simulink model "Microgrid_transition_model_092021"  (R2020a)
settings: Solver=VariableStepAuto  StartTime=0.0  StopTime=10  MaxStep=1e-4  RelTol=1e-3
PreLoadFcn:
  | %run('FC_microgrid_param.m')
  | %load('bat_grid_init.m')
InitFcn:
  | %load myisoModel_init;
  | run('FC_microgrid_param.m')
  | tic
  | run('CARTinitFcn.m')
  | %caseNo = 2;
  | 
  | %if (caseNo == 1)
  | %set_param(['Isolated_grid_paper_model_022521/SignalGen'], 'ActiveScenario', 'PStep222kW');
  | %else
  | %set_param(['Isolated_grid_paper_model_022521/SignalGen'], 'ActiveScenario', 'QStep222kVAr');
  | 
  | %end;
StopFcn:
  | toc
undefined symbols (not defined in the file): breakpoints1, breakpoints2, cp_table_data, ctrl, D1, D11, Delta, DiscIntNeverNeededParam, DT, FC_BESS, find_system, gcbh, libFC_BESS, LowerLimit, magnitude, oversize, pq_ts, sps_rtmsupport, timer, ts, Ts, Ts_APC, Ts_Control, Ts_Power, UpperLimit
libraries: powerlib x128, powerlib_meascontrol x81, simulink x63, powerlib_extras x40, simulink_extras x12, sps_avr x7, pi_ctrl x4, SignalEditorBlockLib x2, libLgBattery x1, libFC_PV x1, eePowerMeasurement x1, spsDieselMotorModel x1
(part 7 of 10)

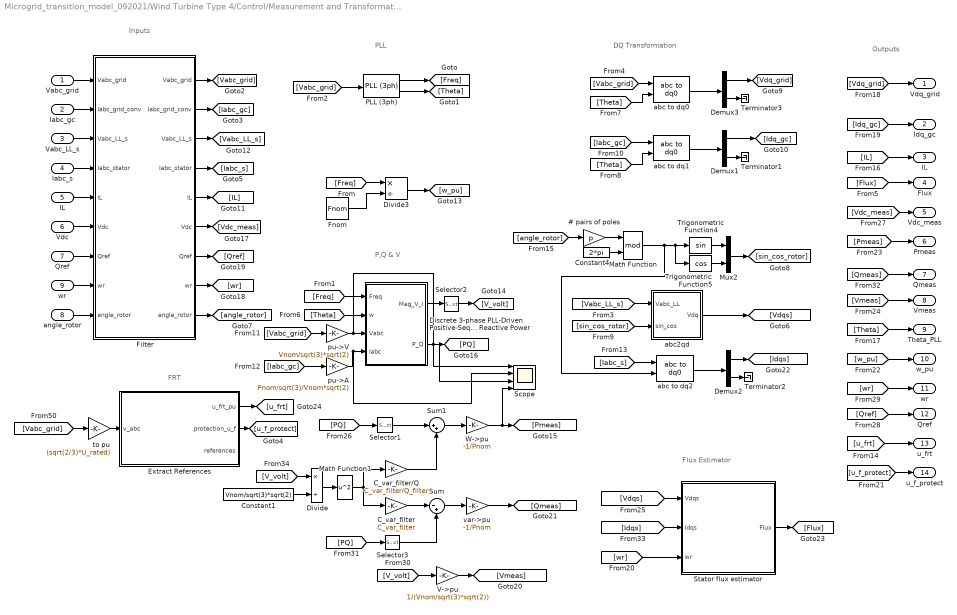
== system Microgrid_transition_model_092021/Wind Turbine Type 4/Control/Measurement and Transformation ==
  note: Flux Estimator
  note: Outputs
  note: PLL
  note: DQ Transformation
  note: P,Q & V
  note: Inputs
  note: FRT
  Vabc_grid : Inport
  Iabc_gc : Inport  Port=2
  Vabc_LL_s : Inport  Port=3
  Iabc_s : Inport  Port=4
  IL : Inport  Port=5
  Vdc : Inport  Port=6
  Qref : Inport  Port=7
  angle_rotor : Inport  Port=8
  wr : Inport  Port=9
  # pairs of poles : Gain  Gain=p  SaturateOnIntegerOverflow=on  OutDataTypeStr=Inherit: Same as input  ParamDataTypeStr=Inherit: Same as input
  C_var_filter : Gain  Gain=C_var_filter  SaturateOnIntegerOverflow=on  OutDataTypeStr=Inherit: Same as input  ParamDataTypeStr=Inherit: Same as input
  C_var_filter/Q : Gain  Gain=C_var_filter/Q_filter  SaturateOnIntegerOverflow=on  OutDataTypeStr=Inherit: Same as input  ParamDataTypeStr=Inherit: Same as input
  Constant1 : Constant  Value=Vnom/sqrt(3)*sqrt(2)
  Constant4 : Constant  Value=2*pi
  Demux1 : Demux  Outputs=[2 1]
      settings: DisplayOption=none
  Demux2 : Demux  Outputs=[2 1]
      settings: DisplayOption=none
  Demux3 : Demux  Outputs=[2 1]
      settings: DisplayOption=none
  Discrete 3-phase PLL-Driven Positive-Sequence Active & Reactive Power : Subsystem  mask(Discrete 3-phase PLL-Driven Positive-Sequence Active & Reactive Power){Finit=Fnom, Fmin=Fnom*45/60, Par_Vinit=[Vnom/sqrt(3)*sqrt(2) 30], Par_Iinit=[Pnom/sqrt(3)/Vnom*sqrt(2) -10], Ts=Ts}
      mask prompts: Finit "Initial frequency (Hz):"; Fmin "Minimum frequency (Hz):"; Par_Vinit "Voltage initial input: [ Mag  Phase(Degrees) ]"; Par_Iinit "Current initial input: [ Mag  Phase(Degrees) ]"; Ts "Sample time:"
      mask help:
      | This discrete block measures the 3-phase active power P and reactive power Q  associated with a periodic set of 3-phase voltages and currents which may contain harmonics. P and Q are calculated by evaluating the fundamental values (positive-sequence) of the input voltages and currents with a running window over one cycle of the specified frequency (port Freq).
      |  Input port "Sin_Cos" (a two-dimension signal) provides the reference frame required for the computation.
      |
      | input 1: must give the frequency of the fundamental (Hz)
      | Input 2: must contain a  [sin(wt)  cos(wt)] two dimension signal , where w is the rotation speed (rad/s) of the reference frame used for the computation..
      | input 3: Vectorized 3-phase  instantaneous voltage (Vabc)
      | input 4: Vectorized 3-phase instantaneous current (Iabc)
      |
      | Output 1: Vector [Mag_V Mag_I] of the fundamental values (Magnitude) of the voltage & current (peak values of the positive-sequence)
      | Output 2: 3-phase PQ measurement vector [P(W) Q (var)] evaluated at the specified frequency. Current flowing into an RL circuit will produce  positive active and reactive powers.
      |
      | For the first cycle of simulation, the outputs are held constant using the values specified by the parameters "Initial input".
      | he value of the parameter "Minimum frequency" is used to determine the buffer size of the "Variable Transport Delay" block found inside this subsystem.
      mask init:
      | power_initmask();
      settings: OpenFcn=power_openblockproxy();
  Divide : Product  Inputs=*/
  Divide3 : Product  Inputs=*/
  Extract References : Subsystem
  Filter : Subsystem  mask{Freq=Freq_filter, Zeta=Zeta_filter, Ts=Ts}
      mask prompts: Freq "Cut-off frequency (Hz):"; Zeta "Damping factor Zeta:"; Ts "Sample time"
  Fnom : Constant  Value=Fnom
  Math Function : Math  Operator=mod  SignedPower=on  SaturateOnIntegerOverflow=on
  Math Function1 : Math  Operator=square  SignedPower=on  SaturateOnIntegerOverflow=on
  Mux2 : Mux  Inputs=2
  PLL (3ph) : powerlib_meascontrol/PLL/PLL (3ph)  Fmin=0.75*Fnom  Par_Init=[-45 Fnom]  ParK=[60 1400 1]  TcD=1e-4  MaxRateChangeFreq=12  FilterCutOffFreq=25  Ts=Ts  AGC=on
      settings: SourceProductBaseCode=MT,PS
  Scope : Scope  NumInputPorts=4
  Selector1 : Selector  InputPortWidth=2  IndexOptions=Index vector (dialog)  Indices=1  OutputSizes=1
  Selector2 : Selector  InputPortWidth=2  IndexOptions=Index vector (dialog)  Indices=1  OutputSizes=1
  Selector3 : Selector  InputPortWidth=2  IndexOptions=Index vector (dialog)  Indices=2  OutputSizes=1
  Stator flux estimator : Subsystem
  Sum : Sum  Inputs=|-+
  Sum1 : Sum  Inputs=|++
  Terminator1 : Terminator
  Terminator2 : Terminator
  Terminator3 : Terminator
  Trigonometric Function4 : Trigonometry
  Trigonometric Function5 : Trigonometry  Operator=cos
  V->pu : Gain  Gain=1/(Vnom/sqrt(3)*sqrt(2))  SaturateOnIntegerOverflow=on  OutDataTypeStr=Inherit: Same as input  ParamDataTypeStr=Inherit: Same as input
  W->pu : Gain  Gain=-1/Pnom  SaturateOnIntegerOverflow=on  OutDataTypeStr=Inherit: Same as input  ParamDataTypeStr=Inherit: Same as input
  abc to dq0 : powerlib_meascontrol/Transformations/abc to dq0  Alignment=90 degrees behind phase A axis
      settings: SourceProductBaseCode=MT,PS
  abc to dq1 : powerlib_meascontrol/Transformations/abc to dq0  Alignment=90 degrees behind phase A axis
      settings: SourceProductBaseCode=MT,PS
  abc to dq2 : powerlib_meascontrol/Transformations/abc to dq0  Alignment=90 degrees behind phase A axis
      settings: SourceProductBaseCode=MT,PS
  abc2qd : Subsystem
  pu->A : Gain  Gain=Pnom/sqrt(3)/Vnom*sqrt(2)  SaturateOnIntegerOverflow=on  OutDataTypeStr=Inherit: Same as input  ParamDataTypeStr=Inherit: Same as input
  pu->V : Gain  Gain=Vnom/sqrt(3)*sqrt(2)  SaturateOnIntegerOverflow=on  OutDataTypeStr=Inherit: Same as input  ParamDataTypeStr=Inherit: Same as input
  to pu : Gain  Gain=(sqrt(2/3)*U_rated)
  "var->pu " : Gain  Gain=-1/Pnom  SaturateOnIntegerOverflow=on  OutDataTypeStr=Inherit: Same as input  ParamDataTypeStr=Inherit: Same as input
  Vdq_grid : Outport  VectorParamsAs1DForOutWhenUnconnected=off
  Idq_gc : Outport  Port=2  VectorParamsAs1DForOutWhenUnconnected=off
  "IL " : Outport  Port=3  VectorParamsAs1DForOutWhenUnconnected=off
  Flux : Outport  Port=4  VectorParamsAs1DForOutWhenUnconnected=off
  Vdc_meas : Outport  Port=5  VectorParamsAs1DForOutWhenUnconnected=off
  Pmeas : Outport  Port=6  VectorParamsAs1DForOutWhenUnconnected=off
  Qmeas : Outport  Port=7  VectorParamsAs1DForOutWhenUnconnected=off
  Vmeas : Outport  Port=8  VectorParamsAs1DForOutWhenUnconnected=off
  Theta_PLL : Outport  Port=9  VectorParamsAs1DForOutWhenUnconnected=off
  w_pu : Outport  Port=10  VectorParamsAs1DForOutWhenUnconnected=off
  "wr " : Outport  Port=11  VectorParamsAs1DForOutWhenUnconnected=off
  "Qref " : Outport  Port=12  VectorParamsAs1DForOutWhenUnconnected=off
  u_frt : Outport  Port=13
  u_f_protect : Outport  Port=14
  wires:
  Filter/9("angle_rotor ") -> [angle_rotor]
  angle_rotor/1 -> Filter/9(angle_rotor)
  Stator flux estimator/1(Flux) -> [Flux]
  # pairs of poles/1 -> Math Function/1
  Constant4/1 -> Math Function/2
  abc2qd/1(Vdq) -> [Vdqs]
  Trigonometric Function5/1 -> Mux2/2
  Trigonometric Function4/1 -> Mux2/1
  [angle_rotor] -> # pairs of poles/1
  [Vabc_LL_s] -> abc2qd/1(Vabc_LL)
  [sin_cos_rotor] -> abc2qd/2(sin_cos)
  Mux2/1 -> [sin_cos_rotor]
  Demux2/1 -> [Idqs]
  Demux2/2 -> Terminator2/1
  abc to dq2/1 -> Demux2/1
  [Iabc_s] -> abc to dq2/1
  [Vdqs] -> Stator flux estimator/1(Vdqs)
  [Idqs] -> Stator flux estimator/2(Idqs)
  [wr] -> Stator flux estimator/3(wr)
  [Qmeas] -> Qmeas/1
  "var->pu "/1 -> [Qmeas]
  [PQ] -> Selector3/1
  V->pu/1 -> [Vmeas]
  [V_volt] -> V->pu/1
  Selector2/1 -> [V_volt]
  Discrete 3-phase PLL-Driven Positive-Sequence Active & Reactive Power/1(Mag_V_I) -> Selector2/1
  Demux1/2 -> Terminator1/1
  Demux3/1 -> [Vdq_grid]
  Demux3/2 -> Terminator3/1
  abc to dq1/1 -> Demux1/1
  abc to dq0/1 -> Demux3/1
  PLL (3ph)/1 -> [Freq]
  Fnom/1 -> Divide3/2
  Divide3/1 -> [w_pu]
  pu->V/1 -> Scope/1, Discrete 3-phase PLL-Driven Positive-Sequence Active & Reactive Power/3(Vabc)
  W->pu/1 -> Scope/4, [Pmeas]
  [Freq] -> Divide3/1
  [Freq] -> Discrete 3-phase PLL-Driven Positive-Sequence Active & Reactive Power/1(Freq)
  PLL (3ph)/2 -> [Theta]
  [Vabc_grid] -> abc to dq0/1
  [Theta] -> Discrete 3-phase PLL-Driven Positive-Sequence Active & Reactive Power/2(w)
  [Theta] -> abc to dq0/2
  [Theta] -> abc to dq1/2
  [Vabc_grid] -> PLL (3ph)/1
  [Iabc_gc] -> abc to dq1/1
  [Theta] -> Theta_PLL/1
  Demux1/1 -> [Idq_gc]
  [Vdq_grid] -> Vdq_grid/1
  [Idq_gc] -> Idq_gc/1
  [w_pu] -> w_pu/1
  [Pmeas] -> Pmeas/1
  [Vmeas] -> Vmeas/1
  pu->A/1 -> Discrete 3-phase PLL-Driven Positive-Sequence Active & Reactive Power/4(Iabc), Scope/2
  [PQ] -> Selector1/1
  [Vdc_meas] -> Vdc_meas/1
  [Qref] -> "Qref "/1
  [wr] -> "wr "/1
  [Flux] -> Flux/1
  [Vabc_grid] -> pu->V/1
  [Iabc_gc] -> pu->A/1
  Discrete 3-phase PLL-Driven Positive-Sequence Active & Reactive Power/2(P_Q) -> Scope/3, [PQ]
  Vabc_grid/1 -> Filter/1(Vabc_grid)
  Vdc/1 -> Filter/6(Vdc)
  Qref/1 -> Filter/7(Qref)
  wr/1 -> Filter/8(wr)
  Filter/1("Vabc_grid ") -> [Vabc_grid]
  Filter/2("Iabc_grid_conv ") -> [Iabc_gc]
  Filter/4("Iabc_stator ") -> [Iabc_s]
  Filter/6("Vdc ") -> [Vdc_meas]
  Filter/8("wr ") -> [wr]
  Filter/7("Qref ") -> [Qref]
  Iabc_gc/1 -> Filter/2(Iabc_grid_conv)
  Iabc_s/1 -> Filter/4(Iabc_stator)
  Vabc_LL_s/1 -> Filter/3(Vabc_LL_s)
  Filter/3("Vabc_LL_s ") -> [Vabc_LL_s]
  [V_volt] -> Divide/1
  Constant1/1 -> Divide/2
  Divide/1 -> Math Function1/1
  Selector3/1 -> Sum/2
  C_var_filter/1 -> Sum/1
  Sum/1 -> "var->pu "/1
  Math Function1/1 -> C_var_filter/Q/1, C_var_filter/1
  Selector1/1 -> Sum1/1
  C_var_filter/Q/1 -> Sum1/2
  Sum1/1 -> W->pu/1
  IL/1 -> Filter/5(IL)
  Filter/5("IL ") -> [IL]
  [IL] -> "IL "/1
  Math Function/1 -> abc to dq2/2, Trigonometric Function5/1, Trigonometric Function4/1
  Extract References/1(u_frt_pu) -> [u_frt]
  Extract References/2(protection_u_f) -> [u_f_protect]
  [Vabc_grid] -> to pu/1
  [u_frt] -> u_frt/1
  [u_f_protect] -> u_f_protect/1
  to pu/1 -> Extract References/1(v_abc)

== system Microgrid_transition_model_092021/Wind Turbine Type 4/Control/Speed & Pitch Control1 ==
  note: Pitch Control
  note: Pitch Compensation
  note: Speed Regulator
  note: Note :
      | This control system is based on the report:
      | Dynamic Modeling of GE 1.5 and 3.6 Wind Turbine-Generators;
      | Prepared by: Nicholas W. Miller, William W. Price, Juan J. Sanchez-Gasca;
      | October 27, 2003, Version 3.0
      | GE-Power Systems Energy Consulting
      | Copyright 2002 General Electric Company, U.S.A.
      |
      | Another reference is:
      |
      | DYNAMIC MODELING OF GE 1.5 AND 3.6 MW WIND TURBINE GENERATORS
      | FOR STABILITY SIMULATIONS
      | Nicholas W. Miller, Juan J. Sanchez-Gasca, William W. Price Robert W. Delmerico
      | GE Power Systems GE Research
      | Schenectady, NY Niskayuna, NY
      |
      | 0-7803-7989-6/03/$17.00 02003 IEEE
  note: Current Regulator
  wr : Inport
  Pmeas : Inport  Port=2
  IL : Inport  Port=3
  Tgain : Inport  Port=4
  Pref : Inport  Port=5
  0-inf : Saturate  UpperLimit=inf  LowerLimit=0
  0-pitch_max : Saturate  UpperLimit=pitch_max  LowerLimit=0
  "0-pitch_max " : Saturate  UpperLimit=pitch_max  LowerLimit=0
  Constant1 : Constant
  Discrete PI Controller1 : Subsystem  DialogController=POWERSYS.PowerSysDialog  mask(Discrete PI Controller){Kp=Kp_compensation, Ki=Ki_compensation, Par_Limits=[pitch_max 0], Init=0, Ts=Ts}
      mask prompts: Kp "Proportional gain (Kp):"; Ki "Integral gain (Ki):"; Par_Limits "Output limits: [ Upper   Lower ]"; Init "Output initial value:"; Ts "Sample time:"
      mask help: This block implements a discrete PI controller.
      mask init:
      | UpperLimit=Par_Limits(1);
      | LowerLimit=Par_Limits(2);
      | power_initmask();
      mask Help: This block is part of a subset of blocks in the Extras library that does not have documentation associated with it, other than the block mask description.
      mask Display: disp('PI');
  Discrete PI Controller2 : Subsystem  DialogController=POWERSYS.PowerSysDialog  mask(Discrete PI Controller){Kp=Kp_boost_cur_reg*1, Ki=Ki_boost_cur_reg*0.005, Par_Limits=[1 0], Init=0.5, Ts=Ts}
      mask prompts: Kp "Proportional gain (Kp):"; Ki "Integral gain (Ki):"; Par_Limits "Output limits: [ Upper   Lower ]"; Init "Output initial value:"; Ts "Sample time:"
      mask help: This block implements a discrete PI controller.
      mask init:
      | UpperLimit=Par_Limits(1);
      | LowerLimit=Par_Limits(2);
      | power_initmask();
      mask Help: This block is part of a subset of blocks in the Extras library that does not have documentation associated with it, other than the block mask description.
      mask Display: disp('PI');
  First-Order Filter : powerlib_meascontrol/Filters/First-Order Filter  FilterType=Lowpass  Tc=Pitch_time_constant  Ts=Ts  Initialize=on  Vac_Init=[0.8 -25 60]*0  Vdc_Init=0  PlotResponse=off  FreqRange="[0,  200,  1]"
      settings: SourceProductBaseCode=MT,PS
  First-Order Filter1 : powerlib_meascontrol/Filters/First-Order Filter  FilterType=Lowpass  Tc=T_speed  Ts=Ts  Initialize=on  Vac_Init=[0, 0, 0]  Vdc_Init=1+init(1)/100  PlotResponse=off  FreqRange="[0,  200,  1]"
      settings: SourceProductBaseCode=MT,PS
  Gain2 : Gain  Gain=Kp_pitch  SaturateOnIntegerOverflow=on  OutDataTypeStr=Inherit: Same as input  ParamDataTypeStr=Inherit: Same as input
  Less Than : RelationalOperator  Operator=<=  OutDataTypeStr=boolean  RndMeth=Simplest
  PID Controller1 : simulink/Continuous/PID Controller  Controller=PI  Form=Parallel  TimeDomain=Discrete-time  UseExternalTs=off  SampleTime=-1  IntegratorMethod=Forward Euler  FilterMethod=Forward Euler  ControllerParametersSource=internal  P=Kp_speed  I=Ki_speed  D=0  UseFilter=on  N=100  TunerSelectOption=Transfer Function Based (PID Tuner App)  InitialConditionSource=internal  InitialConditionForIntegrator=0  InitialConditionForFilter=0  DifferentiatorICPrevScaledInput=0  ExternalReset=none  TrackingMode=off  Kt=1  LimitOutput=on  UpperSaturationLimit=1.  LowerSaturationLimit=0.8  LinearizeAsGain=on  AntiWindupMode=back-calculation  Kb=1e4  POutMin=[]  POutMax=[]  IOutMin=[]  IOutMax=[]  DOutMin=[]  DOutMax=[]  NOutMin=[]  NOutMax=[]  SumOutMin=[]  SumOutMax=[]  SaturationOutMin=[]  SaturationOutMax=[]  PParamMin=[]  PParamMax=[]  IParamMin=[]  IParamMax=[]  DParamMin=[]  DParamMax=[]  NParamMin=[]  NParamMax=[]  KbParamMin=[]  KbParamMax=[]  KtParamMin=[]  KtParamMax=[]  KbOutMin=[]  KbOutMax=[]  KtOutMin=[]  KtOutMax=[]  IntegratorOutMin=[]  IntegratorOutMax=[]  FilterOutMin=[]  FilterOutMax=[]  SumI1OutMin=[]  SumI1OutMax=[]  SumI2OutMin=[]  SumI2OutMax=[]  SumI3OutMin=[]  SumI3OutMax=[]  SumI4OutMin=[]  SumI4OutMax=[]  SumDOutMin=[]  SumDOutMax=[]  DifferentiatorOutMin=[]  DifferentiatorOutMax=[]  FilterDiffOutCoefMin=[]  FilterDiffOutCoefMax=[]  ReciprocalOutMin=[]  ReciprocalOutMax=[]  SumDenOutMin=[]  SumDenOutMax=[]  SumNumOutMin=[]  SumNumOutMax=[]  DivideOutMin=[]  DivideOutMax=[]  UdiffTsProdOutMin=[]  UdiffTsProdOutMax=[]  NTsProdOutMin=[]  NTsProdOutMax=[]  UintegralTsProdOutMin=[]  UintegralTsProdOutMax=[]  UngainTsProdOutMin=[]  UngainTsProdOutMax=[]  IntegratorContinuousStateAttributes=''  IntegratorStateMustResolveToSignalObject=off  IntegratorRTWStateStorageClass=Auto  FilterContinuousStateAttributes=''  FilterStateMustResolveToSignalObject=off  FilterRTWStateStorageClass=Auto  ParallelPVariant=InternalParameters  IdealPVariant=Disabled  IVariant=InternalParameters  DVariant=Disabled  IntegratorVariant=Discrete  SatVariant=Enabled  AWVariant=BackCalculation  PCopyVariant=Disabled  TRVariant=Disabled  FdbkBlocksVariant=Forward  IdealPFdbkVariant=Disabled  SatFdbkVariant=Disabled  DerivativeFilterVariant=Disabled  NVariant=Disabled  NCopyVariant=Disabled_SignalSpec  FilterICVariant=Disabled  IntegratorICVariant=InternalICs  ExternalResetVariant=Disabled  TRSumVariant=Passthrough  SumFdbkVariant=Disabled  SumVariant=Sum_PI  TsampFilterVariant=InternalTs  TsampNgainVariant=Passthrough  TsampIntegralVariant=Passthrough
  Rate Limiter   1 : RateLimiter  RisingSlewLimit=pitch_rate  FallingSlewLimit=-pitch_rate
  Scope : Scope  NumInputPorts=4
  Scope1 : Scope  NumInputPorts=4
  Scope2 : Scope
  Sum : Sum  Inputs=-+  SaturateOnIntegerOverflow=on
  Sum1 : Sum  Inputs=|+-
  Sum2 : Sum  Inputs=|+-  SaturateOnIntegerOverflow=on
  Sum3 : Sum  Inputs=|++
  Sum4 : Sum  Inputs=|+-
  Switch : Switch  Threshold=0.75
  Switch1 : Switch  Criteria=u2 > Threshold  Threshold=0.5
  Tracking Curve : Fcn  Expr=-0.5551*u(1)^2+1.183*u(1)+0.425
  pu_elec->pu_mec : Gain  Gain=Pnom/Pmec
  wref : Constant
  Duty_Cycle : Outport  VectorParamsAs1DForOutWhenUnconnected=off
  Pitch (deg) : Outport  Port=2  VectorParamsAs1DForOutWhenUnconnected=off
  wires:
  wr/1 -> Scope1/2, Sum/2, Sum1/1  "wr"
  0-inf/1 -> pu_elec->pu_mec/1
  pu_elec->pu_mec/1 -> Tracking Curve/1, Sum2/1, Switch/2  "Pmes"
  wref/1 -> Switch/1
  Switch/1 -> First-Order Filter1/1
  Sum1/1 -> PID Controller1/1, Scope1/3  "wdiff"
  Pref/1 -> Sum2/2  "Pref"
  Sum3/1 -> Rate Limiter   1/1
  Rate Limiter   1/1 -> "0-pitch_max "/1
  Gain2/1 -> 0-pitch_max/1
  Discrete PI Controller1/1(Out) -> Sum3/2  "Pitch_comp"
  Pmeas/1 -> 0-inf/1
  0-pitch_max/1 -> Sum3/1  "Pitch_contrl"
  "0-pitch_max "/1 -> First-Order Filter/1
  Sum/1 -> Gain2/1
  First-Order Filter/1 -> Pitch (deg)/1  "Pitch"
  Sum2/1 -> Discrete PI Controller1/1(Error)
  First-Order Filter1/1 -> Scope1/1, Sum1/2, Sum/1  "wref"
  Tracking Curve/1 -> Switch/3
  Sum4/1 -> Discrete PI Controller2/1(Error)
  IL/1 -> Sum4/2, Scope/3  "IL"
  Discrete PI Controller2/1(Out) -> Duty_Cycle/1, Scope/4  "Duty cycle"
  Switch1/1 -> Scope2/1, Sum4/1, Scope/2  "ILref"
  Tgain/1 -> Switch1/3, Less Than/1
  Constant1/1 -> Less Than/2
  Less Than/1 -> Switch1/2
  PID Controller1/1 -> Scope1/4, Switch1/1  "ILref"

== system Microgrid_transition_model_092021/../Control/Excitation Control system/Discrete PI Controller ==
  note: Pierre Giroux, Gilbert Sybille
      | Power System Simulation Laboratory
      | IREQ, Hydro-Quebc
  note: Discrete PID Controller
  Error : Inport  SampleTime=Ts
  Discrete-Time Integrator : DiscreteIntegrator  InitialCondition=Init  SampleTime=Ts  LimitOutput=on  UpperSaturationLimit=UpperLimit  LowerSaturationLimit=LowerLimit  ICPrevOutput=DiscIntNeverNeededParam  ICPrevScaledInput=DiscIntNeverNeededParam
  Kp4 : Gain  Gain=Kp  SaturateOnIntegerOverflow=on  SampleTime=Ts  OutDataTypeStr=Inherit: Same as input  ParamDataTypeStr=Inherit: Same as input
  Kp5 : Gain  Gain=Ki  SaturateOnIntegerOverflow=on  SampleTime=Ts  OutDataTypeStr=Inherit: Same as input  ParamDataTypeStr=Inherit: Same as input
  Saturation2 : Saturate  UpperLimit=UpperLimit  LowerLimit=LowerLimit  SampleTime=Ts
  Sum6 : Sum  InputSameDT=on  SaturateOnIntegerOverflow=on  SampleTime=Ts  OutDataTypeStr=Inherit: Same as first input
  Zero-Order Hold : ZeroOrderHold  SampleTime=Ts
  Out : Outport  SampleTime=Ts  InitialOutput=0  VectorParamsAs1DForOutWhenUnconnected=off
  wires:
  Error/1 -> Kp4/1, Kp5/1
  Sum6/1 -> Saturation2/1
  Kp5/1 -> Discrete-Time Integrator/1
  Kp4/1 -> Zero-Order Hold/1
  Discrete-Time Integrator/1 -> Sum6/2
  Saturation2/1 -> Out/1
  Zero-Order Hold/1 -> Sum6/1

== system Microgrid_transition_model_092021/../Control/Grid-side converter Control system/Discrete PI Controller ==
  note: Pierre Giroux, Gilbert Sybille
      | Power System Simulation Laboratory
      | IREQ, Hydro-Quebc
  note: Discrete PID Controller
  Error : Inport  SampleTime=Ts
  Discrete-Time Integrator : DiscreteIntegrator  InitialCondition=Init  SampleTime=Ts  LimitOutput=on  UpperSaturationLimit=UpperLimit  LowerSaturationLimit=LowerLimit  ICPrevOutput=DiscIntNeverNeededParam  ICPrevScaledInput=DiscIntNeverNeededParam
  Kp4 : Gain  Gain=Kp  SaturateOnIntegerOverflow=on  SampleTime=Ts  OutDataTypeStr=Inherit: Same as input  ParamDataTypeStr=Inherit: Same as input
  Kp5 : Gain  Gain=Ki  SaturateOnIntegerOverflow=on  SampleTime=Ts  OutDataTypeStr=Inherit: Same as input  ParamDataTypeStr=Inherit: Same as input
  Saturation2 : Saturate  UpperLimit=UpperLimit  LowerLimit=LowerLimit  SampleTime=Ts
  Sum6 : Sum  InputSameDT=on  SaturateOnIntegerOverflow=on  SampleTime=Ts  OutDataTypeStr=Inherit: Same as first input
  Zero-Order Hold : ZeroOrderHold  SampleTime=Ts
  Out : Outport  SampleTime=Ts  InitialOutput=0  VectorParamsAs1DForOutWhenUnconnected=off
  wires:
  Error/1 -> Kp4/1, Kp5/1
  Sum6/1 -> Saturation2/1
  Kp5/1 -> Discrete-Time Integrator/1
  Kp4/1 -> Zero-Order Hold/1
  Discrete-Time Integrator/1 -> Sum6/2
  Saturation2/1 -> Out/1
  Zero-Order Hold/1 -> Sum6/1

== system Microgrid_transition_model_092021/../Control/Grid-side converter Control system/Discrete PI Controller1 ==
  note: Pierre Giroux, Gilbert Sybille
      | Power System Simulation Laboratory
      | IREQ, Hydro-Quebc
  note: Discrete PID Controller
  Error : Inport  SampleTime=Ts
  Discrete-Time Integrator : DiscreteIntegrator  InitialCondition=Init  SampleTime=Ts  LimitOutput=on  UpperSaturationLimit=UpperLimit  LowerSaturationLimit=LowerLimit  ICPrevOutput=DiscIntNeverNeededParam  ICPrevScaledInput=DiscIntNeverNeededParam
  Kp4 : Gain  Gain=Kp  SaturateOnIntegerOverflow=on  SampleTime=Ts  OutDataTypeStr=Inherit: Same as input  ParamDataTypeStr=Inherit: Same as input
  Kp5 : Gain  Gain=Ki  SaturateOnIntegerOverflow=on  SampleTime=Ts  OutDataTypeStr=Inherit: Same as input  ParamDataTypeStr=Inherit: Same as input
  Saturation2 : Saturate  UpperLimit=UpperLimit  LowerLimit=LowerLimit  SampleTime=Ts
  Sum6 : Sum  InputSameDT=on  SaturateOnIntegerOverflow=on  SampleTime=Ts  OutDataTypeStr=Inherit: Same as first input
  Zero-Order Hold : ZeroOrderHold  SampleTime=Ts
  Out : Outport  SampleTime=Ts  InitialOutput=0  VectorParamsAs1DForOutWhenUnconnected=off
  wires:
  Error/1 -> Kp4/1, Kp5/1
  Sum6/1 -> Saturation2/1
  Kp5/1 -> Discrete-Time Integrator/1
  Kp4/1 -> Zero-Order Hold/1
  Discrete-Time Integrator/1 -> Sum6/2
  Saturation2/1 -> Out/1
  Zero-Order Hold/1 -> Sum6/1

== system Microgrid_transition_model_092021/../Control/Grid-side converter Control system/INT ==
  note: INTEGRATOR (Trapezoidal) with External limits & Reset & Hold
  Max : Inport
  Min : Inport  Port=2
  In : Inport  Port=3
  Ki : Inport  Port=4
  Hold : Inport  Port=5
  Reset : Inport  Port=6
  Reset Value : Inport  Port=7
  Gain : Gain  Gain=Ts* 0.5  SaturateOnIntegerOverflow=on  OutDataTypeStr=Inherit: Same as input  ParamDataTypeStr=Inherit: Same as input
  IC = 0 : UnitDelay  SampleTime=Ts  HasFrameUpgradeWarning=on
  IC = i_ic : UnitDelay  SampleTime=Ts  HasFrameUpgradeWarning=on
  Logical Operator4 : Logic  Operator=OR
  MinMax : MinMax  Inputs=2  InputSameDT=on  SaturateOnIntegerOverflow=on
  MinMax1 : MinMax  Function=max  Inputs=2  InputSameDT=on  SaturateOnIntegerOverflow=on
  Product : Product  SaturateOnIntegerOverflow=on  OutDataTypeStr=Inherit: Same as first input
  S6 : Subsystem  mask(Limiter with External Limits){}
      mask Display: disp('      Limiter\n')
  Sum : Sum  InputSameDT=on  SaturateOnIntegerOverflow=on  OutDataTypeStr=Inherit: Same as first input
  Sum1 : Sum  InputSameDT=on  SaturateOnIntegerOverflow=on  OutDataTypeStr=Inherit: Same as first input
  Switch2 : Switch  Threshold=0.5  SaturateOnIntegerOverflow=on  InputSameDT=on
  Switch3 : Switch  Threshold=0.5  SaturateOnIntegerOverflow=on  InputSameDT=on
  Switch7 : Switch  Threshold=0.5  SaturateOnIntegerOverflow=on  InputSameDT=on
  Out : Outport  InitialOutput=0  VectorParamsAs1DForOutWhenUnconnected=off
  wires:
  S6/1("  ") -> IC = i_ic/1, Out/1
  Gain/1 -> Product/1
  Sum1/1 -> Product/2
  Ki/1 -> Gain/1
  IC = 0/1 -> Sum1/2
  In/1 -> IC = 0/1, Sum1/1
  Product/1 -> Sum/1
  Sum/1 -> S6/2(In)
  Hold/1 -> Logical Operator4/1
  Reset/1 -> Switch7/2, Logical Operator4/2
  Logical Operator4/1 -> Switch2/2, Switch3/2
  Switch2/1 -> MinMax/1
  Max/1 -> Switch2/3, MinMax/2
  Reset Value/1 -> Switch7/1
  MinMax/1 -> S6/1(MAX)
  MinMax1/1 -> S6/3(MIN)
  Switch3/1 -> MinMax1/1
  Min/1 -> Switch3/3, MinMax1/2
  IC = i_ic/1 -> Switch7/3
  Switch7/1 -> Switch2/1, Sum/2, Switch3/1

== system Microgrid_transition_model_092021/../Control/Measurement and Transformation/Discrete 3-phase PLL-Driven Positive-Sequence Active & Reactive Power ==
  note: Discrete 3-phase PLL-driven Positive-Sequence Active & Reactive Power
  note: Pierre Giroux, Gilbert Sybille
      | Power System Simulation Laboratory
      | IREQ, Hydro-Quebc
  Freq : Inport  PortDimensions=1
  w : Inport  Port=2  PortDimensions=1
  Vabc : Inport  Port=3  PortDimensions=3
  Iabc : Inport  Port=4  PortDimensions=3
  Deg->Rad : Gain  Gain=pi/180  SaturateOnIntegerOverflow=on  OutDataTypeStr=Inherit: Same as input  ParamDataTypeStr=Inherit: Same as input
  Discrete 3-phase PLL-Driven Positive-Sequence Fundamental Value : Subsystem  mask(Discrete 3-phase PLL-Driven Positive-Sequence Fundamental Value){Finit=Finit, Fmin=Fmin, Par_Init=Par_Vinit, Ts=Ts}
      mask prompts: Finit "Initial frequency (Hz):"; Fmin "Minimum frequency (Hz):"; Par_Init "Initial input (positive component): [ Mag  Phase-relative-to-PLL(degrees) ]"; Ts "Sample time:"
      mask help:
      | For a supplied fundamental frequency (port Freq), this discrete block computes  the positive-sequence component (Magnitude and Phase)  of a set of three balanced or unbalanced signals (port abc) which may contain harmonics.
      |  Input port "Sin_Cos" (a two-dimension signal) provides the reference frame required for the computation..
      |  First and second outputs return respectively the magnitude and phase (in degrees relative to the PLL phase)) of the fundamental.
      | For the first cycle of simulation, the outputs are held constant to the values specified by the parameter "Initial input".
      | constant to the values specified by the parameter "Initial input". The value of the parameter "Minimum frequency" is used to determine the buffer size of the "Variable Transport Delay" block found inside this subsystem.
      mask init:
      | Real_Init=Par_Init(1)*cos(pi/180*Par_Init(2));
      | Imag_Init=Par_Init(1)*sin(pi/180*Par_Init(2));
      | power_initmask();
      settings: OpenFcn=power_openblockproxy();
  Discrete 3-phase PLL-Driven Positive-Sequence Fundamental Value2 : Subsystem  mask(Discrete 3-phase PLL-Driven Positive-Sequence Fundamental Value){Finit=Finit, Fmin=Fmin, Par_Init=Par_Iinit, Ts=Ts}
      mask prompts: Finit "Initial frequency (Hz):"; Fmin "Minimum frequency (Hz):"; Par_Init "Initial input (positive component): [ Mag  Phase-relative-to-PLL(degrees) ]"; Ts "Sample time:"
      mask help:
      | For a supplied fundamental frequency (port Freq), this discrete block computes  the positive-sequence component (Magnitude and Phase)  of a set of three balanced or unbalanced signals (port abc) which may contain harmonics.
      |  Input port "Sin_Cos" (a two-dimension signal) provides the reference frame required for the computation..
      |  First and second outputs return respectively the magnitude and phase (in degrees relative to the PLL phase)) of the fundamental.
      | For the first cycle of simulation, the outputs are held constant to the values specified by the parameter "Initial input".
      | constant to the values specified by the parameter "Initial input". The value of the parameter "Minimum frequency" is used to determine the buffer size of the "Variable Transport Delay" block found inside this subsystem.
      mask init:
      | Real_Init=Par_Init(1)*cos(pi/180*Par_Init(2));
      | Imag_Init=Par_Init(1)*sin(pi/180*Par_Init(2));
      | power_initmask();
      settings: OpenFcn=power_openblockproxy();
  Gain1 : Gain  Gain=3/2  SaturateOnIntegerOverflow=on  OutDataTypeStr=Inherit: Same as input  ParamDataTypeStr=Inherit: Same as input
  Mux2 : Mux  Inputs=2
  Mux3 : Mux  Inputs=2
  Product : Product  InputSameDT=on  SaturateOnIntegerOverflow=on  OutDataTypeStr=Inherit: Same as first input
  Product1 : Product  InputSameDT=on  SaturateOnIntegerOverflow=on  OutDataTypeStr=Inherit: Same as first input
  Product2 : Product  InputSameDT=on  SaturateOnIntegerOverflow=on  OutDataTypeStr=Inherit: Same as first input
  Sum : Sum  Inputs=+-  InputSameDT=on  SaturateOnIntegerOverflow=on  OutDataTypeStr=Inherit: Same as first input
  Trigonometric Function : Trigonometry
  Trigonometric Function1 : Trigonometry  Operator=cos
  Mag_V_I : Outport  VectorParamsAs1DForOutWhenUnconnected=off
  P_Q : Outport  Port=2  VectorParamsAs1DForOutWhenUnconnected=off
  wires:
  Vabc/1 -> Discrete 3-phase PLL-Driven Positive-Sequence Fundamental Value/3(abc)
  Freq/1 -> Discrete 3-phase PLL-Driven Positive-Sequence Fundamental Value/1(Freq), Discrete 3-phase PLL-Driven Positive-Sequence Fundamental Value2/1(Freq)
  w/1 -> Discrete 3-phase PLL-Driven Positive-Sequence Fundamental Value/2(w), Discrete 3-phase PLL-Driven Positive-Sequence Fundamental Value2/2(w)
  Discrete 3-phase PLL-Driven Positive-Sequence Fundamental Value/2(Phase) -> Sum/1
  Discrete 3-phase PLL-Driven Positive-Sequence Fundamental Value/1(Mag) -> Mux3/1, Product2/1
  Discrete 3-phase PLL-Driven Positive-Sequence Fundamental Value2/2(Phase) -> Sum/2
  Sum/1 -> Deg->Rad/1
  Deg->Rad/1 -> Trigonometric Function1/1, Trigonometric Function/1
  Trigonometric Function1/1 -> Product/2
  Trigonometric Function/1 -> Product1/1
  Mux2/1 -> Gain1/1
  Product/1 -> Mux2/1
  Product1/1 -> Mux2/2
  Mux3/1 -> Mag_V_I/1
  Gain1/1 -> P_Q/1
  Product2/1 -> Product/1, Product1/2
  Discrete 3-phase PLL-Driven Positive-Sequence Fundamental Value2/1(Mag) -> Mux3/2, Product2/2
  Iabc/1 -> Discrete 3-phase PLL-Driven Positive-Sequence Fundamental Value2/3(abc)

== system Microgrid_transition_model_092021/../Control/Measurement and Transformation/Filter ==
  Vabc_grid : Inport
  Iabc_grid_conv : Inport  Port=2
  Vabc_LL_s : Inport  Port=3
  Iabc_stator : Inport  Port=4
  IL : Inport  Port=5
  Vdc : Inport  Port=6
  Qref : Inport  Port=7
  wr : Inport  Port=8
  angle_rotor : Inport  Port=9
  Second-Order Filter{,1..6} (7 alike) : powerlib_meascontrol/Filters/Second-Order Filter  FilterType=Lowpass  Fo=Freq  Zeta=Zeta  Ts=Ts  Initialize=off  Vac_Init="[0,  0,  60]"  Vdc_Init=0  PlotResponse=off  FreqRange=[0, 500, 1]
      settings: SourceProductBaseCode=MT,PS
  Second-Order Filter7 : powerlib_meascontrol/Filters/Second-Order Filter  FilterType=Lowpass  Fo=Freq  Zeta=Zeta  Ts=Ts  Initialize=on  Vac_Init=[0.8 -25 60]*0  Vdc_Init=Vdc_nom  PlotResponse=off  FreqRange=[0, 500, 1]
      settings: SourceProductBaseCode=MT,PS
  Second-Order Filter8 : powerlib_meascontrol/Filters/Second-Order Filter  FilterType=Lowpass  Fo=Freq  Zeta=Zeta  Ts=Ts  Initialize=on  Vac_Init=[0.8 -25 60]*0  Vdc_Init=1+init(1)/100  PlotResponse=off  FreqRange=[0, 500, 1]
      settings: SourceProductBaseCode=MT,PS
  "Vabc_grid " : Outport  VectorParamsAs1DForOutWhenUnconnected=off
  "Iabc_grid_conv " : Outport  Port=2  VectorParamsAs1DForOutWhenUnconnected=off
  "Vabc_LL_s " : Outport  Port=3  VectorParamsAs1DForOutWhenUnconnected=off
  "Iabc_stator " : Outport  Port=4  VectorParamsAs1DForOutWhenUnconnected=off
  "IL " : Outport  Port=5  VectorParamsAs1DForOutWhenUnconnected=off
  "Vdc " : Outport  Port=6  VectorParamsAs1DForOutWhenUnconnected=off
  "Qref " : Outport  Port=7  VectorParamsAs1DForOutWhenUnconnected=off
  "wr " : Outport  Port=8  VectorParamsAs1DForOutWhenUnconnected=off
  "angle_rotor " : Outport  Port=9  VectorParamsAs1DForOutWhenUnconnected=off
  wires:
  Iabc_stator/1 -> Second-Order Filter3/1
  Second-Order Filter2/1 -> "Vabc_LL_s "/1
  Vabc_LL_s/1 -> Second-Order Filter2/1
  Iabc_grid_conv/1 -> Second-Order Filter1/1
  Vabc_grid/1 -> Second-Order Filter/1
  Second-Order Filter4/1 -> "IL "/1
  IL/1 -> Second-Order Filter4/1
  Second-Order Filter5/1 -> "Qref "/1
  Qref/1 -> Second-Order Filter5/1
  Second-Order Filter8/1 -> "wr "/1
  wr/1 -> Second-Order Filter8/1
  Second-Order Filter3/1 -> "Iabc_stator "/1
  Second-Order Filter7/1 -> "Vdc "/1
  Vdc/1 -> Second-Order Filter7/1
  Second-Order Filter1/1 -> "Iabc_grid_conv "/1
  Second-Order Filter/1 -> "Vabc_grid "/1
  Second-Order Filter6/1 -> "angle_rotor "/1
  angle_rotor/1 -> Second-Order Filter6/1

== system Microgrid_transition_model_092021/../Control/Measurement and Transformation/Stator flux estimator ==
  note: Quasi steady state flux at generator stator
  Vdqs : Inport
  Idqs : Inport  Port=2
  wr : Inport  Port=3
  Divide2 : Product  Inputs=**
  Divide4 : Product  Inputs=*/
  Divide7 : Product  Inputs=**
  Divide8 : Product  Inputs=*/
  First-Order Filter : powerlib_meascontrol/Filters/First-Order Filter  FilterType=Lowpass  Tc=Flux_meas_time_constant  Ts=Ts  Initialize=on  Vac_Init=[0, 0, 0]  Vdc_Init=1  PlotResponse=off  FreqRange="[0,  200,  1]"
      settings: SourceProductBaseCode=MT,PS
  Gain : Gain  Gain=-1
  Magnitude of flux : Fcn  Expr=sqrt(u(1)^2+u(2)^2)
  Mux1 : Mux  Inputs=2
  Rs2 : Constant  Value=Resistance
  Rs4 : Constant  Value=Resistance
  Selector1 : Selector  InputPortWidth=2  IndexOptions=Index vector (dialog)  Indices=2  OutputSizes=1
  Selector3 : Selector  InputPortWidth=2  IndexOptions=Index vector (dialog)  Indices=2  OutputSizes=1
  Selector7 : Selector  InputPortWidth=2  IndexOptions=Index vector (dialog)  Indices=1  OutputSizes=1
  Selector8 : Selector  InputPortWidth=2  IndexOptions=Index vector (dialog)  Indices=1  OutputSizes=1
  Sum2 : Sum  Inputs=|+-
  Sum4 : Sum  Inputs=|+-
  avoid division by 0 : Saturate  UpperLimit=inf  LowerLimit=1e-6
  Flux : Outport  VectorParamsAs1DForOutWhenUnconnected=off
  wires:
  wr/1 -> avoid division by 0/1
  Sum2/1 -> Divide4/1
  Divide4/1 -> Mux1/1  "phi_d"
  Divide2/1 -> Sum2/2  "Rs*Iq"
  Selector1/1 -> Sum2/1  "Vq"
  Rs2/1 -> Divide2/2
  Selector3/1 -> Divide2/1  "Iq"
  Vdqs/1 -> Selector1/1, Selector7/1
  Idqs/1 -> Selector3/1, Selector8/1
  Divide7/1 -> Sum4/2  "Rs*Id"
  Selector7/1 -> Sum4/1  "Vd"
  Rs4/1 -> Divide7/2
  Selector8/1 -> Divide7/1  "Id"
  Sum4/1 -> Divide8/1
  Gain/1 -> Divide8/2
  Divide8/1 -> Mux1/2  "phi_q"
  Mux1/1 -> Magnitude of flux/1
  Magnitude of flux/1 -> First-Order Filter/1
  avoid division by 0/1 -> Divide4/2, Gain/1
  First-Order Filter/1 -> Flux/1

== system Microgrid_transition_model_092021/../Control/Measurement and Transformation/abc2qd ==
  note: This subsystem converts Vab and Vbc to Vd,Vq. The sine and cosine com-
      | puted here are sent to the inverse transformation subsystem qd/abc.
  Vabc_LL : Inport
  sin_cos : Inport  Port=2
  Fcn2 : Fcn  Expr=(u[4]*(2*u[1]+u[2]) + (sqrt(3)*u[2]*u[3])) * 1/3
  Fcn3 : Fcn  Expr=(u[3]*(2*u[1]+u[2]) + (-sqrt(3)*u[2]*u[4])) * 1/3
  Mux : Mux  Inputs=2
  Mux1 : Mux  Inputs=[ 2 2 ]
  Selector : Selector  InputPortWidth=3  IndexOptions=Index vector (dialog)  Indices=[1 2]  OutputSizes=1
  Vdq : Outport  InitialOutput=0  VectorParamsAs1DForOutWhenUnconnected=off
  wires:
  Selector/1 -> Mux1/1
  Mux/1 -> Vdq/1
  sin_cos/1 -> Mux1/2
  Vabc_LL/1 -> Selector/1
  Mux1/1 -> Fcn2/1, Fcn3/1
  Fcn2/1 -> Mux/2
  Fcn3/1 -> Mux/1

== system Microgrid_transition_model_092021/../Control/Speed & Pitch Control/Discrete PI Controller ==
  note: Pierre Giroux, Gilbert Sybille
      | Power System Simulation Laboratory
      | IREQ, Hydro-Quebc
  note: Discrete PID Controller
  Error : Inport  SampleTime=Ts
  Discrete-Time Integrator : DiscreteIntegrator  InitialCondition=Init  SampleTime=Ts  LimitOutput=on  UpperSaturationLimit=UpperLimit  LowerSaturationLimit=LowerLimit  ICPrevOutput=DiscIntNeverNeededParam  ICPrevScaledInput=DiscIntNeverNeededParam
  Kp4 : Gain  Gain=Kp  SaturateOnIntegerOverflow=on  SampleTime=Ts  OutDataTypeStr=Inherit: Same as input  ParamDataTypeStr=Inherit: Same as input
  Kp5 : Gain  Gain=Ki  SaturateOnIntegerOverflow=on  SampleTime=Ts  OutDataTypeStr=Inherit: Same as input  ParamDataTypeStr=Inherit: Same as input
  Saturation2 : Saturate  UpperLimit=UpperLimit  LowerLimit=LowerLimit  SampleTime=Ts
  Sum6 : Sum  InputSameDT=on  SaturateOnIntegerOverflow=on  SampleTime=Ts  OutDataTypeStr=Inherit: Same as first input
  Zero-Order Hold : ZeroOrderHold  SampleTime=Ts
  Out : Outport  SampleTime=Ts  InitialOutput=0  VectorParamsAs1DForOutWhenUnconnected=off
  wires:
  Error/1 -> Kp4/1, Kp5/1
  Sum6/1 -> Saturation2/1
  Kp5/1 -> Discrete-Time Integrator/1
  Kp4/1 -> Zero-Order Hold/1
  Discrete-Time Integrator/1 -> Sum6/2
  Saturation2/1 -> Out/1
  Zero-Order Hold/1 -> Sum6/1

== system Microgrid_transition_model_092021/../Control/Speed & Pitch Control/Discrete PI Controller1 ==
  note: Pierre Giroux, Gilbert Sybille
      | Power System Simulation Laboratory
      | IREQ, Hydro-Quebc
  note: Discrete PID Controller
  Error : Inport  SampleTime=Ts
  Discrete-Time Integrator : DiscreteIntegrator  InitialCondition=Init  SampleTime=Ts  LimitOutput=on  UpperSaturationLimit=UpperLimit  LowerSaturationLimit=LowerLimit  ICPrevOutput=DiscIntNeverNeededParam  ICPrevScaledInput=DiscIntNeverNeededParam
  Kp4 : Gain  Gain=Kp  SaturateOnIntegerOverflow=on  SampleTime=Ts  OutDataTypeStr=Inherit: Same as input  ParamDataTypeStr=Inherit: Same as input
  Kp5 : Gain  Gain=Ki  SaturateOnIntegerOverflow=on  SampleTime=Ts  OutDataTypeStr=Inherit: Same as input  ParamDataTypeStr=Inherit: Same as input
  Saturation2 : Saturate  UpperLimit=UpperLimit  LowerLimit=LowerLimit  SampleTime=Ts
  Sum6 : Sum  InputSameDT=on  SaturateOnIntegerOverflow=on  SampleTime=Ts  OutDataTypeStr=Inherit: Same as first input
  Zero-Order Hold : ZeroOrderHold  SampleTime=Ts
  Out : Outport  SampleTime=Ts  InitialOutput=0  VectorParamsAs1DForOutWhenUnconnected=off
  wires:
  Error/1 -> Kp4/1, Kp5/1
  Sum6/1 -> Saturation2/1
  Kp5/1 -> Discrete-Time Integrator/1
  Kp4/1 -> Zero-Order Hold/1
  Discrete-Time Integrator/1 -> Sum6/2
  Saturation2/1 -> Out/1
  Zero-Order Hold/1 -> Sum6/1

== system Microgrid_transition_model_092021/../Control/Speed & Pitch Control/Discrete PI Controller2 ==
  note: Pierre Giroux, Gilbert Sybille
      | Power System Simulation Laboratory
      | IREQ, Hydro-Quebc
  note: Discrete PID Controller
  Error : Inport  SampleTime=Ts
  Discrete-Time Integrator : DiscreteIntegrator  InitialCondition=Init  SampleTime=Ts  LimitOutput=on  UpperSaturationLimit=UpperLimit  LowerSaturationLimit=LowerLimit  ICPrevOutput=DiscIntNeverNeededParam  ICPrevScaledInput=DiscIntNeverNeededParam
  Kp4 : Gain  Gain=Kp  SaturateOnIntegerOverflow=on  SampleTime=Ts  OutDataTypeStr=Inherit: Same as input  ParamDataTypeStr=Inherit: Same as input
  Kp5 : Gain  Gain=Ki  SaturateOnIntegerOverflow=on  SampleTime=Ts  OutDataTypeStr=Inherit: Same as input  ParamDataTypeStr=Inherit: Same as input
  Saturation2 : Saturate  UpperLimit=UpperLimit  LowerLimit=LowerLimit  SampleTime=Ts
  Sum6 : Sum  InputSameDT=on  SaturateOnIntegerOverflow=on  SampleTime=Ts  OutDataTypeStr=Inherit: Same as first input
  Zero-Order Hold : ZeroOrderHold  SampleTime=Ts
  Out : Outport  SampleTime=Ts  InitialOutput=0  VectorParamsAs1DForOutWhenUnconnected=off
  wires:
  Error/1 -> Kp4/1, Kp5/1
  Sum6/1 -> Saturation2/1
  Kp5/1 -> Discrete-Time Integrator/1
  Kp4/1 -> Zero-Order Hold/1
  Discrete-Time Integrator/1 -> Sum6/2
  Saturation2/1 -> Out/1
  Zero-Order Hold/1 -> Sum6/1

== system Microgrid_transition_model_092021/FC_BESS/SMAInverter/85_SMAControl/InvControl ==
  Uabc : Inport  PortDimensions=3
  Uabc_inv : Inport  Port=2  PortDimensions=3
  Iabc : Inport  Port=3  PortDimensions=3
  cb_stat : Inport  Port=4  OutDataTypeStr=double
  pref : Inport  Port=5
  qref : Inport  Port=6
  fref : Inport  Port=7
  vref : Inport  Port=8
  GF_mode_en : Inport  Port=9
  40_V_Control : Subsystem
  50_I_Control : Subsystem
  Bus Creator : BusCreator  Inputs=11
  Bus Creator1 : BusCreator  Inputs=3
  Bus Selector : BusSelector  OutputSignals=Uabc_ref
  CB_Meas2 : Subsystem
  CB_pu : Subsystem
  CS_controller : Subsystem
  Constant : Constant  Value=0.016666/2.3
  Constant1 : Constant  Value=0.05/2.3
  Constant3 : Constant  Value=0  OutDataTypeStr=boolean
  Constant4 : Constant  OutDataTypeStr=boolean
  Droop : Subsystem
  Goto Tag Visibility1 : GotoTagVisibility  GotoTag=inputs
  Goto Tag Visibility10 : GotoTagVisibility  GotoTag=I_Ctrl
  Goto Tag Visibility2 : GotoTagVisibility  GotoTag=cb_meas
  Goto Tag Visibility4 : GotoTagVisibility  GotoTag=droop
  Goto Tag Visibility5 : GotoTagVisibility  GotoTag=inverter
  Goto Tag Visibility6 : GotoTagVisibility  GotoTag=cb_pu
  Goto Tag Visibility7 : GotoTagVisibility  GotoTag=pll
  Goto Tag Visibility8 : GotoTagVisibility  GotoTag=ref_lim
  Goto Tag Visibility9 : GotoTagVisibility  GotoTag=V_Ctrl
  PLL : Subsystem
  Ref_Limiting : Subsystem
  Uabc_ref : Outport  VectorParamsAs1DForOutWhenUnconnected=off
  tag scope: inputs=scoped
  wires:
  Constant1/1 -> Bus Creator/10  "VQ_droop"
  cb_stat/1 -> Bus Creator/6  "cb_status"
  Uabc/1 -> Bus Creator/1  "Uabc"
  Bus Creator/1 -> [inputs]
  vref/1 -> Bus Creator/8  "vref"
  [inverter] -> Bus Selector/1
  Iabc/1 -> Bus Creator/3  "Iabc"
  fref/1 -> Bus Creator/7  "fref"
  Bus Selector/1 -> Uabc_ref/1  "<Uabc_ref>"
  Constant3/1 -> Bus Creator1/3  "Reset"
  Constant4/1 -> Bus Creator1/2  "Enable"
  GF_mode_en/1 -> Bus Creator1/1  "GF_mode"
  Bus Creator1/1 -> Bus Creator/11  "Control_Word"
  Constant/1 -> Bus Creator/9  "FP_droop"
  qref/1 -> Bus Creator/5  "qref"
  pref/1 -> Bus Creator/4  "pref"
  Uabc_inv/1 -> Bus Creator/2  "Uabc_inv"

== system Microgrid_transition_model_092021/Grid Feeder Protective Relay/R25 - Sync Check v0.1/Phase_Comparator/WrapPi ==
  In1 : Inport
  Compare To Constant1 : simulink/Logic and Bit Operations/Compare To Constant  relop=<=  const=-pi  OutDataTypeStr=boolean
  Compare To Constant2 : simulink/Logic and Bit Operations/Compare To Constant  relop=>=  const=pi  OutDataTypeStr=boolean
  Gain1 : Gain  Gain=2*pi
  Gain2 : Gain  Gain=2*pi
  Sum : Sum  Inputs=++-
  Out1 : Outport
  wires:
  Compare To Constant2/1 -> Gain2/1
  Compare To Constant1/1 -> Gain1/1
  In1/1 -> Sum/2, Compare To Constant1/1, Compare To Constant2/1
  Gain2/1 -> Sum/3
  Gain1/1 -> Sum/1
  Sum/1 -> Out1/1

== system Microgrid_transition_model_092021/Grid Feeder Protective Relay1/R25 - Sync Check v0.1/Phase_Comparator/WrapPi ==
  In1 : Inport
  Compare To Constant1 : simulink/Logic and Bit Operations/Compare To Constant  relop=<=  const=-pi  OutDataTypeStr=boolean
  Compare To Constant2 : simulink/Logic and Bit Operations/Compare To Constant  relop=>=  const=pi  OutDataTypeStr=boolean
  Gain1 : Gain  Gain=2*pi
  Gain2 : Gain  Gain=2*pi
  Sum : Sum  Inputs=++-
  Out1 : Outport
  wires:
  Sum/1 -> Out1/1
  Gain1/1 -> Sum/1
  Gain2/1 -> Sum/3
  In1/1 -> Compare To Constant2/1, Compare To Constant1/1, Sum/2
  Compare To Constant1/1 -> Gain1/1
  Compare To Constant2/1 -> Gain2/1

== system Microgrid_transition_model_092021/Wind Turbine Type 4/APC (atomic)1/Inertial Response (to df)/FBIC ==
  wg (pu) : Inport
  Freq (Hz)1 : Inport  Port=2
  Act1 : Inport  Port=3
  Discrete Transfer Fcn : DiscreteTransferFcn  Numerator=[0.99985 -0.99985]  Denominator=[1 -0.99985]
  Display3 : Display
  Display4 : Display
  FBIC performance1 : Scope  NumInputPorts=2
  Logical Operator1 : Logic  Operator=NOT  AllPortsSameDT=off  OutDataTypeStr=boolean
  Low-Pass Filter 1 : eeGeneralControl/Low-Pass Filter (Discrete or Continuous)  K=1  T=1  B=inf  A=-inf  init_option=Inherited from block input  x0=0  Ts=-1
  Nominal F1 : Constant
  S&H1 : Subsystem  mask{ic=0}
      mask prompts: ic "Initial condition"
  Saturation1 : Saturate  UpperLimit=0.3  LowerLimit=0
  Sum1 : Sum  Inputs=+-|
  adaptive FBIC1 : MATLAB Function  TreatAsAtomicUnit=on
  inertial1 : simulink/Discrete/Discrete Derivative  gainval=1.0  ICPrevScaledInput=1  OutMin=[]  OutMax=[]  OutDataType=fixdt(1, 16)  OutScaling=2^-10  DoSatur=off
  to pu 1 : Gain  Gain=1/60
  Delta_P FBIC1 : Outport
  wires:
  inertial1/1 -> adaptive FBIC1/1(F_de), Display3/1
  adaptive FBIC1/3(P_dr) -> FBIC performance1/2
  adaptive FBIC1/2(P_de) -> FBIC performance1/1
  Freq (Hz)1/1 -> to pu 1/1
  S&H1/1(Out) -> adaptive FBIC1/3(Wi)
  Act1/1 -> adaptive FBIC1/4(Act), Logical Operator1/1
  wg (pu)/1 -> S&H1/1(In)
  adaptive FBIC1/1(Delta_P) -> Saturation1/1
  Logical Operator1/1 -> S&H1/2(S)
  Low-Pass Filter 1/1 -> inertial1/1, Display4/1
  Nominal F1/1 -> Sum1/2
  Saturation1/1 -> Delta_P FBIC1/1
  Sum1/1 -> Discrete Transfer Fcn/1
  to pu 1/1 -> Sum1/1, Low-Pass Filter 1/1
  Discrete Transfer Fcn/1 -> adaptive FBIC1/2(F_dr)

== system Microgrid_transition_model_092021/Wind Turbine Type 4/APC (atomic)1/Inertial Response (to df)/Lock2 ==
  I : Inport
  R : Inport  Port=2
  Constant7 : Constant  Value=0
  Display1 : Display
  Display16 : Display
  Freq Act : Switch  Threshold=0.5
  Logical Operator1 : Logic  Operator=NOT  AllPortsSameDT=off  OutDataTypeStr=boolean
  Logical Operator3 : Logic  Operator=NOT  AllPortsSameDT=off  OutDataTypeStr=boolean
  S&H : Subsystem  mask{ic=0}
      mask prompts: ic "Initial condition"
  Unit Delay : UnitDelay  SampleTime=-1  HasFrameUpgradeWarning=on
  O : Outport
  wires:
  Logical Operator1/1 -> Freq Act/2, Display16/1
  R/1 -> Logical Operator1/1
  Constant7/1 -> Freq Act/3
  Freq Act/1 -> Logical Operator3/1
  S&H/1(Out) -> O/1, Display1/1, Freq Act/1
  I/1 -> S&H/1(In)
  Logical Operator3/1 -> Unit Delay/1
  Unit Delay/1 -> S&H/2(S)

== system Microgrid_transition_model_092021/Wind Turbine Type 4/APC (atomic)1/Inertial Response (to df)/TLIC ==
  Act : Inport
  Delay1 : Delay  DelayLength=1  InitialCondition=0
  Delay2 : Delay  DelayLength=1  InitialCondition=0
  Delay3 : Delay  DelayLength=1  InitialCondition=0
  Display1 : Display
  Display2 : Display
  Scope : Scope  NumInputPorts=4
  adaptive TLIC : MATLAB Function  TreatAsAtomicUnit=on
  Delta_P TLIC : Outport
  wires:
  Delay3/1 -> Scope/2, adaptive TLIC/1("recharge ")  "recharge"
  Delay2/1 -> adaptive TLIC/2("trecharge "), Scope/3  "trecharge"
  Delay1/1 -> adaptive TLIC/3("tIR "), Scope/4  "tIR"
  adaptive TLIC/4(tIR) -> Delay1/1
  adaptive TLIC/3(trecharge) -> Delay2/1
  adaptive TLIC/2(recharge) -> Delay3/1
  Act/1 -> adaptive TLIC/4(Act), Display2/1
  adaptive TLIC/1(Delta_P) -> Delta_P TLIC/1, Display1/1, Scope/1  "dP"

== system Microgrid_transition_model_092021/Wind Turbine Type 4/Control/Excitation Control system/Discrete PI Controller ==
  note: Discrete PID Controller
  note: Pierre Giroux, Gilbert Sybille
      | Power System Simulation Laboratory
      | IREQ, Hydro-Quebc
  Error : Inport  SampleTime=Ts
  Discrete-Time Integrator : DiscreteIntegrator  InitialCondition=Init  SampleTime=Ts  LimitOutput=on  UpperSaturationLimit=UpperLimit  LowerSaturationLimit=LowerLimit  ICPrevOutput=DiscIntNeverNeededParam  ICPrevScaledInput=DiscIntNeverNeededParam
  Kp4 : Gain  Gain=Kp  SaturateOnIntegerOverflow=on  SampleTime=Ts  OutDataTypeStr=Inherit: Same as input  ParamDataTypeStr=Inherit: Same as input
  Kp5 : Gain  Gain=Ki  SaturateOnIntegerOverflow=on  SampleTime=Ts  OutDataTypeStr=Inherit: Same as input  ParamDataTypeStr=Inherit: Same as input
  Saturation2 : Saturate  UpperLimit=UpperLimit  LowerLimit=LowerLimit  SampleTime=Ts
  Sum6 : Sum  InputSameDT=on  SaturateOnIntegerOverflow=on  SampleTime=Ts  OutDataTypeStr=Inherit: Same as first input
  Zero-Order Hold : ZeroOrderHold  SampleTime=Ts
  Out : Outport  SampleTime=Ts  InitialOutput=0  VectorParamsAs1DForOutWhenUnconnected=off
  wires:
  Zero-Order Hold/1 -> Sum6/1
  Saturation2/1 -> Out/1
  Discrete-Time Integrator/1 -> Sum6/2
  Kp4/1 -> Zero-Order Hold/1
  Kp5/1 -> Discrete-Time Integrator/1
  Sum6/1 -> Saturation2/1
  Error/1 -> Kp5/1, Kp4/1

== system Microgrid_transition_model_092021/Wind Turbine Type 4/Control/Grid-Side Inverter Control/Counter AST ==
  Trigger : TriggerPort  VariantControl=Variant  PortDimensions=1
  Constant : Constant
  Memory : Memory  InheritSampleTime=on
  Sum : Sum  Inputs=|++
  Count : Outport
  wires:
  Constant/1 -> Sum/2
  Sum/1 -> Memory/1, Count/1
  Memory/1 -> Sum/1
